simulink model "TwoTanks_FO_2018a"  (R2018a)
settings: Solver=ode4  StartTime=0.0  StopTime=tfinal  FixedStep=dt  RelTol=1e-3  EnableMultiTasking=on
values from neighbouring files (symbols this model uses):
  a1 = 0.0190125110732    [GWO_workspace.mat]    (also in NGWO_TwoTanks_FO.m; SBAIN_2TANKS.m; TwoTanks_FO_main.m; TwoTanks_NL_main.m)
  a2 = 0.594107643424    [GWO_workspace.mat]    (also in NGWO_TwoTanks_FO.m = num2/den2; SBAIN_2TANKS.m = num2/den2; TwoTanks_FO_main.m = num2/den2; TwoTanks_NL_main.m = num2/den2)
  a3 = 0.0893725569407    [GWO_workspace.mat]    (also in NGWO_TwoTanks_FO.m = num3/den3; SBAIN_2TANKS.m = num3/den3; TwoTanks_FO_main.m = num3/den3; TwoTanks_NL_main.m = num3/den3)
  a4 = 0.0670294177055    [GWO_workspace.mat]    (also in NGWO_TwoTanks_FO.m = num4/den4; SBAIN_2TANKS.m = num4/den4; TwoTanks_FO_main.m = num4/den4; TwoTanks_NL_main.m = num4/den4)
  h10 = 0.25    [GWO_workspace.mat]    (also in NGWO_TwoTanks_FO.m; SBAIN_2TANKS.m; TwoTanks_FO_main.m; TwoTanks_NL_main.m)
  H1max = 1    [GWO_workspace.mat]    (also in NGWO_TwoTanks_FO.m; SBAIN_2TANKS.m; TwoTanks_FO_main.m; TwoTanks_NL_main.m)
  h20 = 0.25    [GWO_workspace.mat]    (also in NGWO_TwoTanks_FO.m; SBAIN_2TANKS.m; TwoTanks_FO_main.m; TwoTanks_NL_main.m)
  H2max = 1    [GWO_workspace.mat]    (also in NGWO_TwoTanks_FO.m; SBAIN_2TANKS.m; TwoTanks_FO_main.m; TwoTanks_NL_main.m)
  K0 = 0.525796662699    [GWO_workspace.mat]    (also in NGWO_TwoTanks_FO.m = x(p,1); SBAIN_2TANKS.m = sol(1); TwoTanks_FO_main.m = P1(1,3); resultado_semi_ideal.mat = 0.73123128782)
  K1 = 1.64876894102    [GWO_workspace.mat]    (also in NGWO_TwoTanks_FO.m = x(p,2); SBAIN_2TANKS.m = sol(2); TwoTanks_FO_main.m = P1(1,2); resultado_semi_ideal.mat = 1.78819501719)
settings Model: Creator=joniram  LastModifiedBy=joniram-XPS
settings DataIOCC: ExternalInput=[limV1F_sup, limV1F_inf, limV2F_sup, limV2F_inf]  LimitDataPoints=on  SaveFormat=Array  SignalLoggingSaveFormat=ModelDataLogs
settings OptimizationCC: ExpressionDepthLimit=2147483647  LifeSpan=inf
settings DebuggingCC: UnderspecifiedInitializationDetection=Classic  MergeDetectMultiDrivingBlocksExec=none  SolverPrmCheckMsg=warning  FcnCallInpInsideContextMsg=warning  StateNameClashWarn=warning  SFUnexpectedBacktrackingDiag=warning  SFNoUnconditionalDefaultTransitionDiag=warning  SFExecutionAtInitializationDiag=none
settings HardwareCC: ProdBitPerPointer=32  ProdBitPerSizeT=32  ProdBitPerPtrDiffT=32  ProdLargestAtomicFloat=None  ProdIntDivRoundTo=Undefined  ProdEndianess=Unspecified  ProdWordSize=32  ProdHWDeviceType=32-bit Generic
settings ModelReferenceCC: PropagateSignalLabelsOutOfModel=off
settings CodeAppCC: StateflowObjectComments=on
settings GRTTargetCC: TargetLangStandard=C89/C90 (ANSI)  GeneratePreprocessorConditionals=Disable all  CombineOutputUpdateFcns=off  GRTInterface=on
settings ConfigComp: CovMetricSettings=dw  CovHtmlReporting=on  CovSaveCumulativeToWorkspaceVar=on  CovSaveSingleToWorkspaceVar=on  CovExternalEMLEnable=off

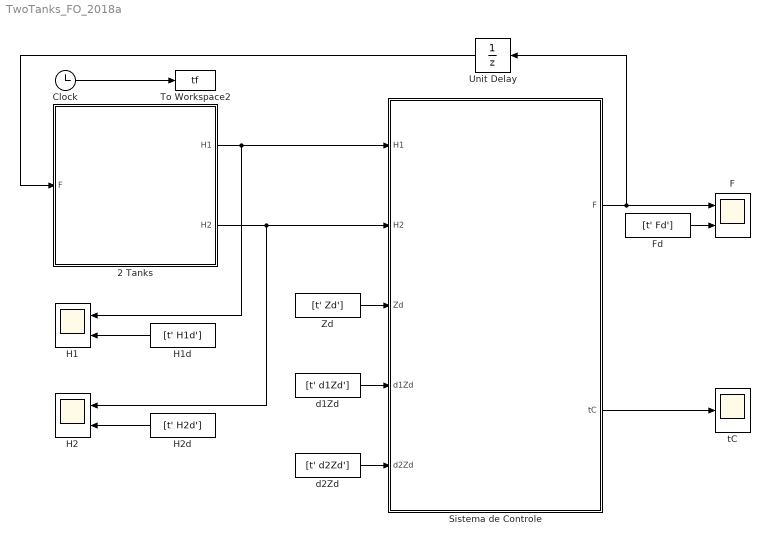
== system TwoTanks_FO_2018a ==
  2 Tanks : Subsystem
  Clock : Clock
  F : Scope  NumInputPorts=2
  Fd : FromWorkspace  VariableName=[t' Fd']  SampleTime=0  OutputAfterFinalValue=Holding final value
  H1 : Scope  NumInputPorts=2
  H1d : FromWorkspace  VariableName=[t' H1d']  SampleTime=0  OutputAfterFinalValue=Holding final value
  H2 : Scope  NumInputPorts=2
  H2d : FromWorkspace  VariableName=[t' H2d']  SampleTime=0  OutputAfterFinalValue=Holding final value
  Sistema de Controle : MATLAB Function  TreatAsAtomicUnit=on
  To Workspace2 : ToWorkspace  VariableName=tf  SampleTime=-1
  Unit Delay : UnitDelay  SampleTime=-1  HasFrameUpgradeWarning=on
  Zd : FromWorkspace  VariableName=[t' Zd']  SampleTime=0  OutputAfterFinalValue=Holding final value
  d1Zd : FromWorkspace  VariableName=[t' d1Zd']  SampleTime=0  OutputAfterFinalValue=Holding final value
  d2Zd : FromWorkspace  VariableName=[t' d2Zd']  SampleTime=0  OutputAfterFinalValue=Holding final value
  tC : Scope
  wires:
  2 Tanks/2(H2) -> Sistema de Controle/2(H2), H2/1
  2 Tanks/1(H1) -> Sistema de Controle/1(H1), H1/1
  d2Zd/1 -> Sistema de Controle/5(d2Zd)
  Zd/1 -> Sistema de Controle/3(Zd)
  d1Zd/1 -> Sistema de Controle/4(d1Zd)
  Sistema de Controle/1(F) -> F/1, Unit Delay/1
  Sistema de Controle/2(tC) -> tC/1
  Unit Delay/1 -> 2 Tanks/1(F)
  H2d/1 -> H2/2
  Clock/1 -> To Workspace2/1
  H1d/1 -> H1/2
  Fd/1 -> F/2

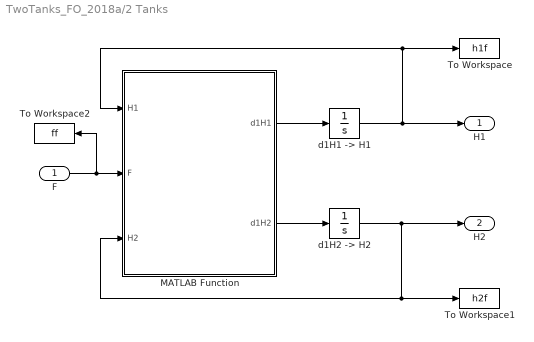
== system TwoTanks_FO_2018a/2 Tanks ==
  F : Inport
  MATLAB Function : MATLAB Function  TreatAsAtomicUnit=on
  To Workspace : ToWorkspace  VariableName=h1f  SampleTime=-1
  To Workspace1 : ToWorkspace  VariableName=h2f  SampleTime=-1
  To Workspace2 : ToWorkspace  VariableName=ff  SampleTime=-1
  "d1H1 -> H1" : Integrator  InitialCondition=h10  LimitOutput=on  UpperSaturationLimit=H1max  LowerSaturationLimit=0
  "d1H2 -> H2" : Integrator  InitialCondition=h20  LimitOutput=on  UpperSaturationLimit=H2max  LowerSaturationLimit=0
  H1 : Outport
  H2 : Outport  Port=2
  wires:
  MATLAB Function/1(d1H1) -> "d1H1 -> H1"/1
  "d1H1 -> H1"/1 -> H1/1, To Workspace/1, MATLAB Function/1(H1)
  MATLAB Function/2(d1H2) -> "d1H2 -> H2"/1
  F/1 -> To Workspace2/1, MATLAB Function/2(F)
  "d1H2 -> H2"/1 -> H2/1, To Workspace1/1, MATLAB Function/3(H2)

== matlab function TwoTanks_FO_2018a/Sistema de Controle ==
  data: F output; tC output; H1 input; H2 input; K1 parameter; K0 parameter; Zd input; d1Zd input; d2Zd input; a1 parameter; a2 parameter; a3 parameter; a4 parameter
function [F, tC] = Controle_Flatness(H1, H2, K1, K0, Zd, d1Zd, d2Zd, a1, a2, a3, a4)
 
  % Gerando Z e d1Z
    Z = H2;
    d1Z = a3*(sqrt(H1)/(H2^2)) - a4/(H2^1.5);
    
  % Termo de Correção em Malha Fechada
    tC = d2Zd - K1*(d1Z - d1Zd) - K0*(Z - Zd); 
    
  % Gerando a expressão final para os controladores
    F = ((2*Z^(5/2)*a4 + 2*Z^4*d1Z)/(a1*a3^2))*tC + (a4^2*d1Z + 4*H2^3*d1Z^3 + 5*Z^(3/2)*a4*d1Z^2 + a2*a3^2*((Z*(a4 + Z^(3/2)*d1Z)^2)/a3^2)^(1/2))/(a1*a3^2);
 
  % Saturação dos Sinais de Controle
    limF_sup = 90; limF_inf = 10;
    F = min(limF_sup, max(limF_inf, F));

== matlab function TwoTanks_FO_2018a/2 Tanks/MATLAB Function ==
  data: H1 input; F input; d1H1 output; H2 input; d1H2 output; a1 parameter; a2 parameter; a3 parameter; a4 parameter
function [d1H1, d1H2] = TwoTanks(H1, F, H2, a1, a2, a3, a4)
  
  % Sistema Dinâmico
    d1H1 = a1*F - a2*sqrt(H1);
    
    d1H2 = a3*(sqrt(H1)/(H2^2)) - a4*(1/(H2^1.5));
